simulink model "Monod_delay_Controller"  (R2020b)
settings: Solver=FixedStepAuto  StartTime=0.0  StopTime=constants.tend  FixedStep=constants.dt  RelTol=1e-3
undefined symbols (not defined in the file or in its folder): constants
libraries: pid_lib x2
settings Model: Creator=newpo  LastModifiedBy=newpo
settings DataIOCC: ReturnWorkspaceOutputs=off

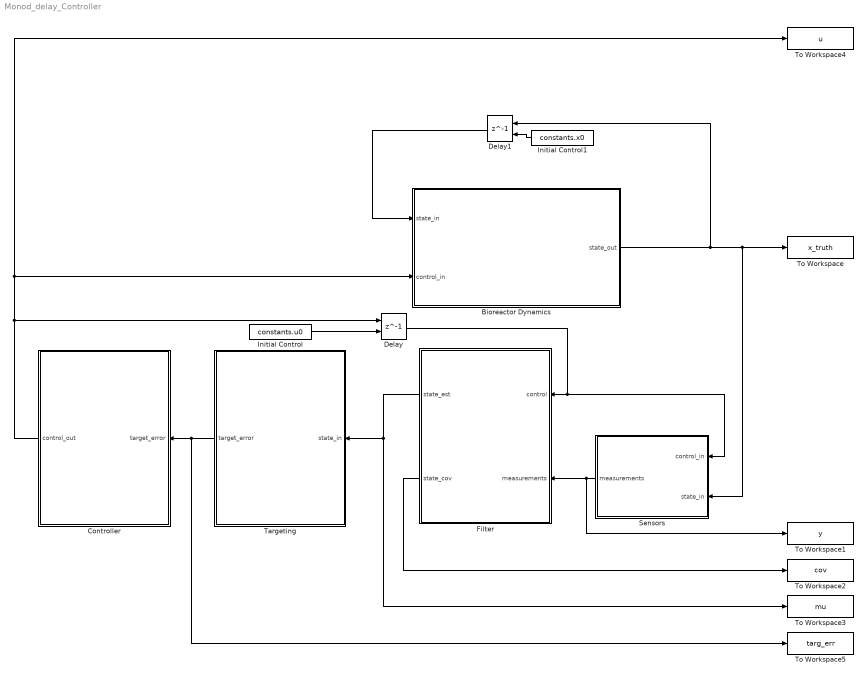
== system Monod_delay_Controller ==
  Bioreactor Dynamics : Subsystem
  Controller : Subsystem
  Delay : Delay  DelayLength=1  InitialConditionSource=Input port  InitialCondition=[constants.w;0;0;constants.Fg]
      settings: InputPortMap=u0,p4
  Delay1 : Delay  DelayLength=1  InitialConditionSource=Input port  InitialCondition=[constants.w;0;0;constants.Fg]
      settings: InputPortMap=u0,p4
  Filter : Subsystem
  Initial Control : Constant  Value=constants.u0
  Initial Control1 : Constant  Value=constants.x0
  Sensors : Subsystem
  Targeting : Subsystem
  To Workspace : ToWorkspace  VariableName=x_truth  SampleTime=-1
  To Workspace1 : ToWorkspace  VariableName=y  SampleTime=-1
  To Workspace2 : ToWorkspace  VariableName=cov  SampleTime=-1
  To Workspace3 : ToWorkspace  VariableName=mu  SampleTime=-1
  To Workspace4 : ToWorkspace  VariableName=u  SampleTime=-1
  To Workspace5 : ToWorkspace  VariableName=targ_err  SampleTime=-1
  wires:
  Bioreactor Dynamics/1(state_out) -> Delay1/1, Sensors/2(state_in), To Workspace/1
  Sensors/1(measurements) -> To Workspace1/1, Filter/2(measurements)
  Filter/1(state_est) -> To Workspace3/1, Targeting/1(state_in)
  Controller/1(control_out) -> To Workspace4/1, Bioreactor Dynamics/2(control_in), Delay/1
  Targeting/1(target_error) -> To Workspace5/1, Controller/1(target_error)
  Filter/2(state_cov) -> To Workspace2/1
  Delay/1 -> Sensors/1(control_in), Filter/1(control)
  Initial Control/1 -> Delay/2
  Delay1/1 -> Bioreactor Dynamics/1(state_in)
  Initial Control1/1 -> Delay1/2

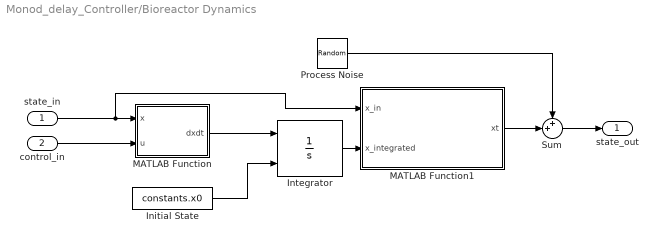
== system Monod_delay_Controller/Bioreactor Dynamics ==
  state_in : Inport
  control_in : Inport  Port=2
  Initial State : Constant  Value=constants.x0
  Integrator : Integrator  InitialConditionSource=external  LimitOutput=on  LowerSaturationLimit=0
  MATLAB Function : MATLAB Function  TreatAsAtomicUnit=on
  MATLAB Function1 : MATLAB Function  TreatAsAtomicUnit=on
  Process Noise : RandomNumber  Variance=diag(constants.Q)  SampleTime=constants.dt
  Sum : Sum  Inputs=++|
  state_out : Outport
  wires:
  Initial State/1 -> Integrator/2
  Sum/1 -> state_out/1
  Process Noise/1 -> Sum/1
  state_in/1 -> MATLAB Function1/1(x_in), MATLAB Function/1(x)
  control_in/1 -> MATLAB Function/2(u)
  MATLAB Function/1(dxdt) -> Integrator/1
  MATLAB Function1/1(xt) -> Sum/2
  Integrator/1 -> MATLAB Function1/2(x_integrated)

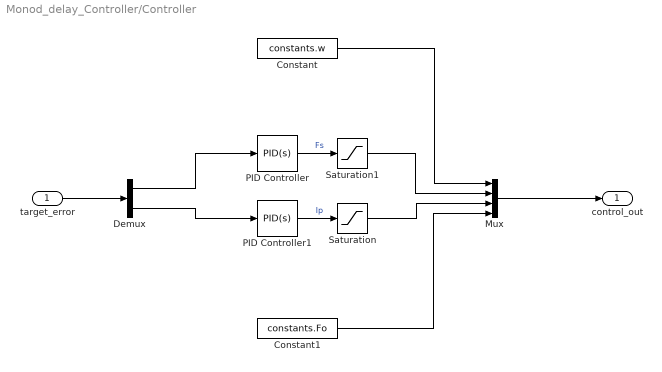
== system Monod_delay_Controller/Controller ==
  target_error : Inport
  Constant : Constant  Value=constants.w
  Constant1 : Constant  Value=constants.Fo
  Demux : Demux  Outputs=2
  Mux : Mux
  PID Controller : pid_lib/PID Controller  Controller=PID  Form=Parallel  TimeDomain=Continuous-time  UseExternalTs=off  SampleTime=-1  IntegratorMethod=Forward Euler  FilterMethod=Forward Euler  ControllerParametersSource=internal  P=constants.Fs_PID(1)  I=constants.Fs_PID(2)  D=constants.Fs_PID(3)  UseFilter=on  N=100  TunerSelectOption=Transfer Function Based (PID Tuner App)  InitialConditionSource=internal  InitialConditionForIntegrator=0  InitialConditionForFilter=0  DifferentiatorICPrevScaledInput=0  ExternalReset=none  TrackingMode=off  Kt=1  LimitOutput=off  SatLimitsSource=internal  UpperSaturationLimit=inf  LowerSaturationLimit=-inf  LinearizeAsGain=on  AntiWindupMode=none  Kb=1  POutMin=[]  POutMax=[]  IOutMin=[]  IOutMax=[]  DOutMin=[]  DOutMax=[]  NOutMin=[]  NOutMax=[]  SumOutMin=[]  SumOutMax=[]  SaturationOutMin=[]  SaturationOutMax=[]  PParamMin=[]  PParamMax=[]  IParamMin=[]  IParamMax=[]  DParamMin=[]  DParamMax=[]  NParamMin=[]  NParamMax=[]  KbParamMin=[]  KbParamMax=[]  KtParamMin=[]  KtParamMax=[]  KbOutMin=[]  KbOutMax=[]  KtOutMin=[]  KtOutMax=[]  IntegratorOutMin=[]  IntegratorOutMax=[]  FilterOutMin=[]  FilterOutMax=[]  SumI1OutMin=[]  SumI1OutMax=[]  SumI2OutMin=[]  SumI2OutMax=[]  SumI3OutMin=[]  SumI3OutMax=[]  SumI4OutMin=[]  SumI4OutMax=[]  SumDOutMin=[]  SumDOutMax=[]  DifferentiatorOutMin=[]  DifferentiatorOutMax=[]  FilterDiffOutCoefMin=[]  FilterDiffOutCoefMax=[]  ReciprocalOutMin=[]  ReciprocalOutMax=[]  SumDenOutMin=[]  SumDenOutMax=[]  SumNumOutMin=[]  SumNumOutMax=[]  DivideOutMin=[]  DivideOutMax=[]  UdiffTsProdOutMin=[]  UdiffTsProdOutMax=[]  NTsProdOutMin=[]  NTsProdOutMax=[]  UintegralTsProdOutMin=[]  UintegralTsProdOutMax=[]  UngainTsProdOutMin=[]  UngainTsProdOutMax=[]  IntegratorContinuousStateAttributes=''  IntegratorStateMustResolveToSignalObject=off  IntegratorRTWStateStorageClass=Auto  FilterContinuousStateAttributes=''  FilterStateMustResolveToSignalObject=off  FilterRTWStateStorageClass=Auto  ParallelPVariant=InternalParameters  IdealPVariant=Disabled  IVariant=InternalParameters  DVariant=InternalParameters  IntegratorVariant=Continuous  SatVariant=Disabled  AWVariant=Passthrough  PCopyVariant=Disabled  TRVariant=Disabled  FdbkBlocksVariant=Forward  IdealPFdbkVariant=Disabled  SatFdbkVariant=Disabled  DerivativeFilterVariant=ContFilter  NVariant=InternalParameters  NCopyVariant=Disabled  FilterICVariant=InternalICsFilter  IntegratorICVariant=InternalICs  ExternalResetVariant=Disabled  TRSumVariant=Passthrough  SumFdbkVariant=Disabled  SumVariant=Sum_PID  TsampFilterVariant=InternalTs  TsampNgainVariant=Passthrough  TsampIntegralVariant=Passthrough  ExternalSaturationOutDataTypeStr=Inherit: Same as second input
  PID Controller1 : pid_lib/PID Controller  Controller=PID  Form=Parallel  TimeDomain=Continuous-time  UseExternalTs=off  SampleTime=-1  IntegratorMethod=Forward Euler  FilterMethod=Forward Euler  ControllerParametersSource=internal  P=constants.IP_PID(1)  I=constants.IP_PID(2)  D=constants.IP_PID(3)  UseFilter=on  N=20  TunerSelectOption=Transfer Function Based (PID Tuner App)  InitialConditionSource=internal  InitialConditionForIntegrator=0  InitialConditionForFilter=0  DifferentiatorICPrevScaledInput=0  ExternalReset=none  TrackingMode=off  Kt=1  LimitOutput=off  SatLimitsSource=internal  UpperSaturationLimit=inf  LowerSaturationLimit=-inf  LinearizeAsGain=on  AntiWindupMode=none  Kb=1  POutMin=[]  POutMax=[]  IOutMin=[]  IOutMax=[]  DOutMin=[]  DOutMax=[]  NOutMin=[]  NOutMax=[]  SumOutMin=[]  SumOutMax=[]  SaturationOutMin=[]  SaturationOutMax=[]  PParamMin=[]  PParamMax=[]  IParamMin=[]  IParamMax=[]  DParamMin=[]  DParamMax=[]  NParamMin=[]  NParamMax=[]  KbParamMin=[]  KbParamMax=[]  KtParamMin=[]  KtParamMax=[]  KbOutMin=[]  KbOutMax=[]  KtOutMin=[]  KtOutMax=[]  IntegratorOutMin=[]  IntegratorOutMax=[]  FilterOutMin=[]  FilterOutMax=[]  SumI1OutMin=[]  SumI1OutMax=[]  SumI2OutMin=[]  SumI2OutMax=[]  SumI3OutMin=[]  SumI3OutMax=[]  SumI4OutMin=[]  SumI4OutMax=[]  SumDOutMin=[]  SumDOutMax=[]  DifferentiatorOutMin=[]  DifferentiatorOutMax=[]  FilterDiffOutCoefMin=[]  FilterDiffOutCoefMax=[]  ReciprocalOutMin=[]  ReciprocalOutMax=[]  SumDenOutMin=[]  SumDenOutMax=[]  SumNumOutMin=[]  SumNumOutMax=[]  DivideOutMin=[]  DivideOutMax=[]  UdiffTsProdOutMin=[]  UdiffTsProdOutMax=[]  NTsProdOutMin=[]  NTsProdOutMax=[]  UintegralTsProdOutMin=[]  UintegralTsProdOutMax=[]  UngainTsProdOutMin=[]  UngainTsProdOutMax=[]  IntegratorContinuousStateAttributes=''  IntegratorStateMustResolveToSignalObject=off  IntegratorRTWStateStorageClass=Auto  FilterContinuousStateAttributes=''  FilterStateMustResolveToSignalObject=off  FilterRTWStateStorageClass=Auto  ParallelPVariant=InternalParameters  IdealPVariant=Disabled  IVariant=InternalParameters  DVariant=InternalParameters  IntegratorVariant=Continuous  SatVariant=Disabled  AWVariant=Passthrough  PCopyVariant=Disabled  TRVariant=Disabled  FdbkBlocksVariant=Forward  IdealPFdbkVariant=Disabled  SatFdbkVariant=Disabled  DerivativeFilterVariant=ContFilter  NVariant=InternalParameters  NCopyVariant=Disabled  FilterICVariant=InternalICsFilter  IntegratorICVariant=InternalICs  ExternalResetVariant=Disabled  TRSumVariant=Passthrough  SumFdbkVariant=Disabled  SumVariant=Sum_PID  TsampFilterVariant=InternalTs  TsampNgainVariant=Passthrough  TsampIntegralVariant=Passthrough  ExternalSaturationOutDataTypeStr=Inherit: Same as second input
  Saturation : Saturate  UpperLimit=constants.Ip_max  LowerLimit=-constants.Ip_max
  Saturation1 : Saturate  UpperLimit=constants.Fs_max  LowerLimit=0
  control_out : Outport
  wires:
  Mux/1 -> control_out/1
  target_error/1 -> Demux/1
  PID Controller/1 -> Saturation1/1  "Fs"
  Demux/1 -> PID Controller/1
  Constant/1 -> Mux/1
  Constant1/1 -> Mux/4
  PID Controller1/1 -> Saturation/1  "Ip"
  Demux/2 -> PID Controller1/1
  Saturation/1 -> Mux/3
  Saturation1/1 -> Mux/2

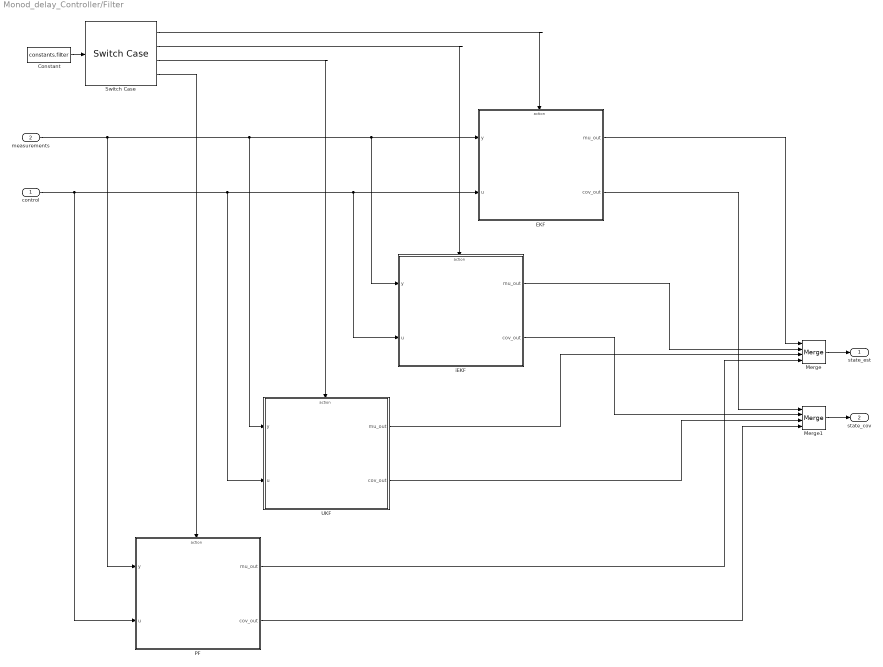
== system Monod_delay_Controller/Filter ==
  control : Inport
  measurements : Inport  Port=2
  Constant : Constant  Value=constants.filter
  EKF : Subsystem  TreatAsAtomicUnit=on
  Merge : Merge  Inputs=4
  Merge1 : Merge  Inputs=4
  PF : Subsystem  TreatAsAtomicUnit=on
  Switch Case : SwitchCase  CaseConditions={FilterTypes.EKF,FilterTypes.iEKF,FilterTypes.UKF,FilterTypes.PF}  ShowDefaultCase=off
  UKF : Subsystem  TreatAsAtomicUnit=on
  iEKF : Subsystem  TreatAsAtomicUnit=on
  state_est : Outport
  state_cov : Outport  Port=2
  wires:
  measurements/1 -> PF/1(y), UKF/1(y), EKF/1(y), iEKF/1(y)
  control/1 -> PF/2(u), UKF/2(u), EKF/2(u), iEKF/2(u)
  EKF/2(cov_out) -> Merge1/1
  Switch Case/1 -> EKF/Action
  Switch Case/2 -> iEKF/Action
  EKF/1(mu_out) -> Merge/1
  iEKF/1(mu_out) -> Merge/2
  Merge/1 -> state_est/1
  Merge1/1 -> state_cov/1
  iEKF/2(cov_out) -> Merge1/2
  Constant/1 -> Switch Case/1
  Switch Case/3 -> UKF/Action
  UKF/1(mu_out) -> Merge/3
  UKF/2(cov_out) -> Merge1/3
  Switch Case/4 -> PF/Action
  PF/2(cov_out) -> Merge1/4
  PF/1(mu_out) -> Merge/4

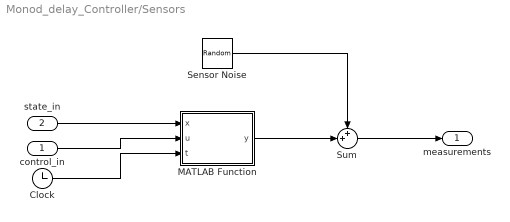
== system Monod_delay_Controller/Sensors ==
  control_in : Inport
  state_in : Inport  Port=2
  Clock : Clock
  MATLAB Function : MATLAB Function  TreatAsAtomicUnit=on
  Sensor Noise : RandomNumber  Variance=diag(constants.R)  SampleTime=constants.dt
  Sum : Sum  Inputs=++|
  measurements : Outport
  wires:
  state_in/1 -> MATLAB Function/1(x)
  control_in/1 -> MATLAB Function/2(u)
  MATLAB Function/1(y) -> Sum/2
  Sum/1 -> measurements/1
  Sensor Noise/1 -> Sum/1
  Clock/1 -> MATLAB Function/3(t)

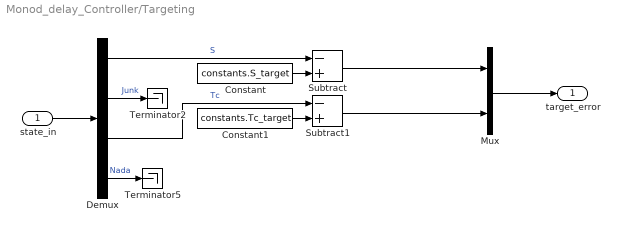
== system Monod_delay_Controller/Targeting ==
  state_in : Inport
  Constant : Constant  Value=constants.S_target
  Constant1 : Constant  Value=constants.Tc_target
  Demux : Demux  Outputs=[1 2 1 -1]
  Mux : Mux  Inputs=2
  Subtract : Sum  Inputs=-+
  Subtract1 : Sum  Inputs=-+
  Terminator2 : Terminator
  Terminator5 : Terminator
  target_error : Outport
  wires:
  state_in/1 -> Demux/1
  Demux/1 -> Subtract/1  "S"
  Constant/1 -> Subtract/2
  Constant1/1 -> Subtract1/2
  Subtract/1 -> Mux/1
  Subtract1/1 -> Mux/2
  Mux/1 -> target_error/1
  Demux/2 -> Terminator2/1  "Junk"
  Demux/4 -> Terminator5/1  "Nada"
  Demux/3 -> Subtract1/1  "Tc"

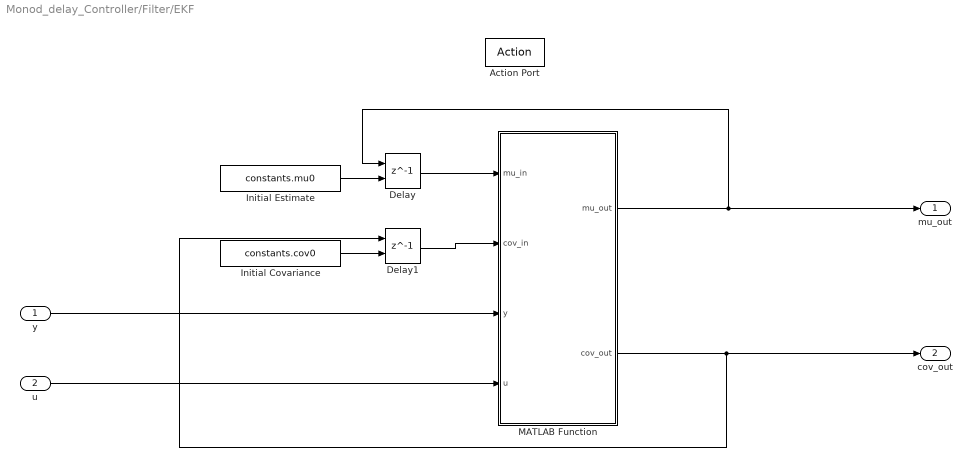
== system Monod_delay_Controller/Filter/EKF ==
  y : Inport
  u : Inport  Port=2
  Action Port : ActionPort  ActionPortLabel=case [ EKF ]:
  Delay : Delay  DelayLength=1  InitialConditionSource=Input port  InitialCondition=0
      settings: InputPortMap=u0,p4
  Delay1 : Delay  DelayLength=1  InitialConditionSource=Input port  InitialCondition=0
      settings: InputPortMap=u0,p4
  Initial Covariance : Constant  Value=constants.cov0
  Initial Estimate : Constant  Value=constants.mu0
  MATLAB Function : MATLAB Function  TreatAsAtomicUnit=on
  mu_out : Outport
  cov_out : Outport  Port=2
  wires:
  y/1 -> MATLAB Function/3(y)
  Initial Estimate/1 -> Delay/2
  Delay1/1 -> MATLAB Function/2(cov_in)
  MATLAB Function/2(cov_out) -> cov_out/1, Delay1/1
  Initial Covariance/1 -> Delay1/2
  u/1 -> MATLAB Function/4(u)
  MATLAB Function/1(mu_out) -> mu_out/1, Delay/1
  Delay/1 -> MATLAB Function/1(mu_in)

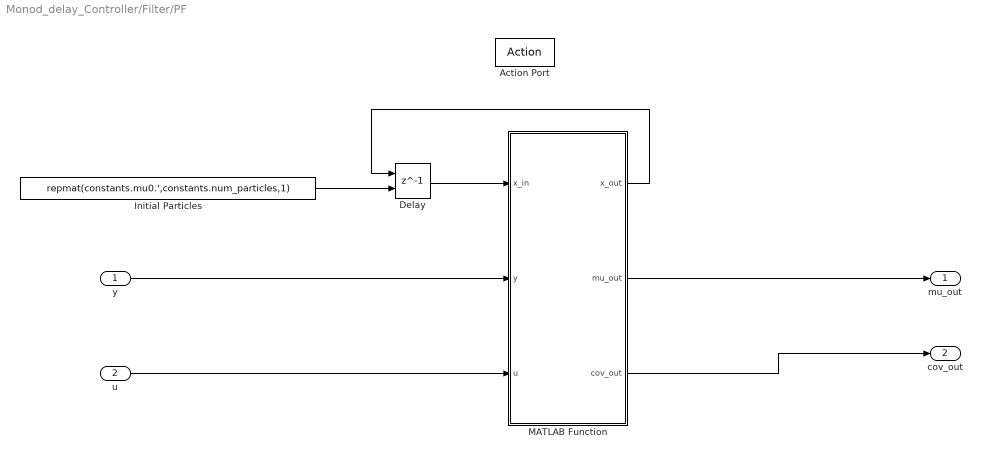
== system Monod_delay_Controller/Filter/PF ==
  y : Inport
  u : Inport  Port=2
  Action Port : ActionPort  ActionPortLabel=case [ PF ]:
  Delay : Delay  DelayLength=1  InitialConditionSource=Input port  InitialCondition=0
      settings: InputPortMap=u0,p4
  Initial Particles : Constant  Value=repmat(constants.mu0.',constants.num_particles,1)
  MATLAB Function : MATLAB Function  TreatAsAtomicUnit=on
  mu_out : Outport
  cov_out : Outport  Port=2
  wires:
  y/1 -> MATLAB Function/2(y)
  MATLAB Function/3(cov_out) -> cov_out/1
  u/1 -> MATLAB Function/3(u)
  MATLAB Function/2(mu_out) -> mu_out/1
  Delay/1 -> MATLAB Function/1(x_in)
  MATLAB Function/1(x_out) -> Delay/1
  Initial Particles/1 -> Delay/2

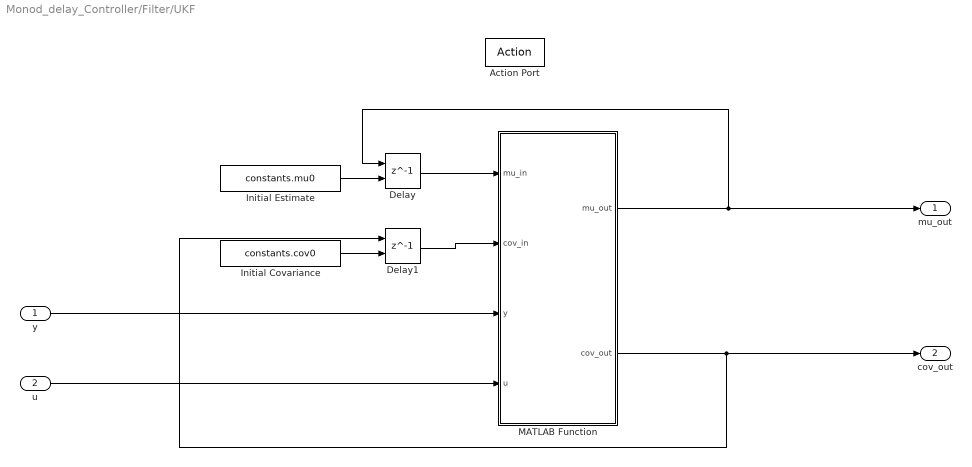
== system Monod_delay_Controller/Filter/UKF ==
  y : Inport
  u : Inport  Port=2
  Action Port : ActionPort  ActionPortLabel=case [ UKF ]:
  Delay : Delay  DelayLength=1  InitialConditionSource=Input port  InitialCondition=0
      settings: InputPortMap=u0,p4
  Delay1 : Delay  DelayLength=1  InitialConditionSource=Input port  InitialCondition=0
      settings: InputPortMap=u0,p4
  Initial Covariance : Constant  Value=constants.cov0
  Initial Estimate : Constant  Value=constants.mu0
  MATLAB Function : MATLAB Function  TreatAsAtomicUnit=on
  mu_out : Outport
  cov_out : Outport  Port=2
  wires:
  y/1 -> MATLAB Function/3(y)
  Initial Estimate/1 -> Delay/2
  Delay1/1 -> MATLAB Function/2(cov_in)
  MATLAB Function/2(cov_out) -> cov_out/1, Delay1/1
  Initial Covariance/1 -> Delay1/2
  u/1 -> MATLAB Function/4(u)
  MATLAB Function/1(mu_out) -> mu_out/1, Delay/1
  Delay/1 -> MATLAB Function/1(mu_in)

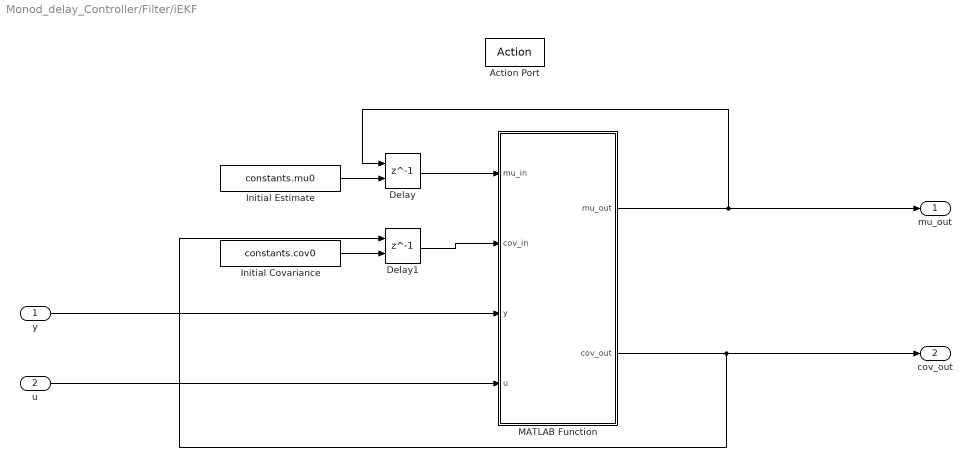
== system Monod_delay_Controller/Filter/iEKF ==
  y : Inport
  u : Inport  Port=2
  Action Port : ActionPort  ActionPortLabel=case [ iEKF ]:
  Delay : Delay  DelayLength=1  InitialConditionSource=Input port  InitialCondition=0
      settings: InputPortMap=u0,p4
  Delay1 : Delay  DelayLength=1  InitialConditionSource=Input port  InitialCondition=0
      settings: InputPortMap=u0,p4
  Initial Covariance : Constant  Value=constants.cov0
  Initial Estimate : Constant  Value=constants.mu0
  MATLAB Function : MATLAB Function  TreatAsAtomicUnit=on
  mu_out : Outport
  cov_out : Outport  Port=2
  wires:
  y/1 -> MATLAB Function/3(y)
  Initial Estimate/1 -> Delay/2
  Delay1/1 -> MATLAB Function/2(cov_in)
  MATLAB Function/2(cov_out) -> cov_out/1, Delay1/1
  Initial Covariance/1 -> Delay1/2
  u/1 -> MATLAB Function/4(u)
  MATLAB Function/1(mu_out) -> mu_out/1, Delay/1
  Delay/1 -> MATLAB Function/1(mu_in)

== matlab function Monod_delay_Controller/Filter/iEKF/MATLAB Function ==
  data: mu_in input; cov_in input; y input; u input; mu_out output; cov_out output; constants parameter
function [mu_out, cov_out] = Monod_iEKF(mu_in, cov_in, y, u, constants)
    % Collect inputs
%     S = mu_in(1); % cell concentration, g/l
%     C = mu_in(2); % substrate concentration, g/l
%     QO2 = mu_in(3); % OTR = OUR, moles/sec
%     Tc = mu_in(4); % Temperature of culture
%     Tinf = mu_in(5); % Temperature of environment
%     V = mu_in(6); % Volume of tank
    mygrowthrate = mu(mu_in(1),mu_in(2)); 
    
    % Collect controls
    w = u(1); % agitator speed, rpm
    Fs = u(2); % substrate feed rate, L/s
    Ip = u(3); % Peltier current, amps
    Fg = u(4); % air feed rate, SLPS
    kLa = w^(1.7)/(Fg^0.1); % kLa coeff
    
    % Collect measurements
%     mf_out = y(1);
%     DO = y(2);
%     Tc_meas = y(3);
%     Tinf_meas = y(4);

    y_end = length(y);
    if y(end) < -1
       y_end = 5; 
    end
    
    % EKF Update
    mu_p = f(mu_in);
    At = A(mu_in);
    cov_p = At*cov_in*(At.') + constants.Q;
    
    % iEKF iteration
    iter_max = 2500; % max number of iterations
    tol = 1E-5;
    n = 0;
    mu_pred = mu_p; % hold the original prediction step mean
    mu_i = mu_p;
    while n < iter_max
        % calculate matrices from previous state
        Ct = C(mu_i); Ct = Ct(1:y_end,:); % update using last time step
        Kt = cov_p*(Ct.')/(Ct*cov_p*(Ct.')+constants.R(1:y_end,1:y_end)); % Kalman gain, using new Ct
        z = g(mu_i);
        z = y(1:y_end) - z(1:y_end);
        mu_i = mu_pred + Kt*(z + Ct*(mu_i - mu_pred));
        err = norm(mu_i - mu_p);
        if err < tol % check convergence between previous step and updated
            break;
        end
        mu_p = mu_i;
        n = n + 1;
    end
    
    Ct = C(mu_i); Ct = Ct(1:y_end,:);
    Kt = cov_p*(Ct.')/(Ct*cov_p*(Ct.')+constants.R(1:y_end,1:y_end)); % Kalman gain
    mu_out = mu_i;
    cov_out = (eye(length(mu_in)) - Kt*Ct)*cov_p;
    
    function xt = f(x)
       xt = zeros(size(x));
       
       xt(1) = x(1) + constants.dt*((constants.S0-x(1))*Fs/x(6)- mygrowthrate/constants.Yxs - constants.m*x(2)); % S = substrate conc
       xt(2) = x(2) + constants.dt*(-Fs/x(6)*x(2)+mygrowthrate); % C = cell conc
       xt(3) = x(3); % QO2 = OUR coefficient
       xt(4) = x(4) + constants.dt/constants.C_heat/x(6)*(constants.N_power*(w^3)+constants.Kq*x(3)*x(2)+(constants.Pp*Ip+(Ip^2)*constants.Rp)*constants.Np + constants.hA*(x(4)-x(5))); % Tc = culture temp
       xt(5) = x(5); % Tinf = environment temp
       xt(6) = x(6) + constants.dt*Fs;
       xt(7:8) = x(1:2);
       if constants.sample_interval > 1
           for i = 2:constants.sample_interval 
               xt(2*i+5:2*i+6) = x(2*i+3:2*i+4); % delayed states
           end
       end
    end
    function At = A(x)
        At = zeros(length(x));
        mymu = mu(x(1),x(2));
        dmu = constants.mu_max*x(2)*constants.Ki*(constants.Ki*constants.Ks-(x(1)^2))/((constants.Ki+x(1))^2)/((constants.Ks+x(1))^2);
        At(1,1) = 1 + constants.dt*(-Fs/x(6)-dmu/constants.Yxs);
        At(1,2) = -constants.dt*mymu - constants.m;
        At(1,6) = -constants.dt*(constants.S0-x(1))*Fs/(x(6)^2);
        At(2,1) = constants.dt*(-Fs/x(6) + dmu);
        At(2,2) = 1 - constants.dt*Fs/x(6) + constants.dt*mymu ;
        At(2,6) = constants.dt*Fs*x(2)/(x(6)^2);
        At(3,3) = 1;
        At(4,2) = constants.dt/constants.C_heat/x(6)*constants.Kq*x(3);
        At(4,3) = constants.dt/constants.C_heat/x(6)*constants.Kq*x(2);
        At(4,4) = 1 + constants.dt/constants.C_heat/x(6)*constants.hA;
        At(4,5) = -constants.dt/constants.C_heat/x(6)*constants.hA;
        At(4,6) = -constants.dt/constants.C_heat/(x(6)^2)*(constants.N_power*(w^3)+constants.Kq*x(3)*x(2)+(constants.Pp*Ip+(Ip^2)*constants.Rp)*constants.Np + constants.hA*(x(4)-x(5))); 
        At(5,5) = 1;
        At(6,6) = 1;
        At(7:8,1:2) = eye(2);
        if constants.sample_interval > 1
           for i = 2:constants.sample_interval 
               At(2*i+5:2*i+6,2*i+3:2*i+4) = eye(2); % delayed states
           end
        end
    end
    function ypred = g(x)
        ypred = zeros(length(y),1);
        ypred(1) = constants.mf_in - x(3)*x(2)/Fg; % Measured mass fraction of O2 leaving system
        ypred(2) = 1 - 1/constants.mf_in*(1/Fg - 1/kLa/constants.pr)*x(3)*x(2); % Measured DO2
        ypred(3) = x(4); % Measured Tc
        ypred(4) = x(5); % measured Tinf
        ypred(5) = x(6);  % measured volume
        ypred(6:7) = x(end-1:end); % last two items in x are the most delayed
    end
    function Ct = C(x)
       Ct = zeros(length(y),length(x));
       Ct(1,2) = -x(3)/Fg;
       Ct(1,3) = -x(2)/Fg;
       Ct(2,2) = -1/constants.mf_in * (1/Fg - 1/constants.pr/kLa)*x(3);
       Ct(2,3) = -1/constants.mf_in * (1/Fg - 1/constants.pr/kLa)*x(2);
       Ct(3,4) = 1;
       Ct(4,5) = 1;
       Ct(5,6) = 1;
       Ct(6,end-1) = 1; % last two items in x are the most delayed
       Ct(7,end) = 1;
    end
    function mut = mu(S,C)
        mut = constants.mu_max*constants.Ki*S/(constants.Ki+S)/(constants.Ks+S)*C ;
    end
end

== matlab function Monod_delay_Controller/Bioreactor Dynamics/MATLAB Function ==
  data: x input; u input; dxdt output; constants parameter
function dxdt = statedot(x,u,constants)
    dxdt = zeros(size(x));
    w = u(1); % agitator speed
    Fs = u(2); % substrate feed rate
    Ip = u(3); % Peltier currents
    mu = constants.mu_max*x(2)*constants.Ki*x(1)/(constants.Ki+x(1))/(constants.Ks+x(1));
    dxdt(1) = constants.S0*Fs/x(6) - Fs/x(6)*x(1) - mu/constants.Yxs - constants.m*x(2); % S = substrate conc
    dxdt(2) = -Fs/x(6)*x(2) + mu; % C = cell conc
    dxdt(3) = 0; % QO2 = OUR coefficient
    dxdt(4) = 1/constants.C_heat/x(6)*(constants.N_power*(w^3)+constants.Kq*x(3)*x(2)+(constants.Pp*Ip+(Ip^2)*constants.Rp)*constants.Np + constants.hA*(x(4)-x(5))); % Tc = culture temp
    dxdt(5) = 0; % Tinf = environment temp
    dxdt(6) = Fs;
    dxdt(7:end) = 0; % these are updated after integration
end

== matlab function Monod_delay_Controller/Sensors/MATLAB Function ==
  data: x input; u input; t input; y output; constants parameter
function y = g(x,u,t,constants)
    y = zeros(7,1);
    w = u(1);
    Fg = u(4);
    kLa = (w^1.7)/(Fg^0.1);
    y(1) = constants.mf_in - x(3)*x(2)/Fg; % Measured mass fraction of O2 leaving system
    y(2) = 1 - 1/constants.mf_in*(1/Fg - 1/kLa/constants.pr)*x(3)*x(2); % Measured DO2
    y(3) = x(4); % Measured Tc
    y(4) = x(5); % measured Tinf
    y(5) = x(6); % measured volume
    if floor(t/constants.dt) > 0 && mod(floor(t/constants.dt),constants.sample_interval)==0
       y(6:7) = x(end-1:end); % last two measurements are delayed by sample_interval
    else
       y(6:7) = [-100; -100]; % throw in bullshit to indicate no major sample 
    end
end

== matlab function Monod_delay_Controller/Filter/EKF/MATLAB Function ==
  data: mu_in input; cov_in input; y input; u input; mu_out output; cov_out output; constants parameter
function [mu_out, cov_out] = Monod_EKF(mu_in, cov_in, y, u, constants)
    % Collect inputs
%     S = mu_in(1); % cell concentration, g/l
%     C = mu_in(2); % substrate concentration, g/l
%     QO2 = mu_in(3); % OTR = OUR, moles/sec
%     Tc = mu_in(4); % Temperature of culture
%     Tinf = mu_in(5); % Temperature of environment
%     V = mu_in(6); % Volume of tank
    mygrowthrate = mu(mu_in(1),mu_in(2)); 
    
    % Collect controls
    w = u(1); % agitator speed, rpm
    Fs = u(2); % substrate feed rate, L/s
    Ip = u(3); % Peltier current, amps
    Fg = u(4); % air feed rate, SLPS
    kLa = w^(1.7)/(Fg^0.1); % kLa coeff
    
    % Collect measurements
%     mf_out = y(1);
%     DO = y(2);
%     Tc_meas = y(3);
%     Tinf_meas = y(4);

    y_end = length(y);
    if y(end) < -1
       y_end = 5; 
    end
    
    % EKF Update
    mu_p = f(mu_in);
    At = A(mu_in);
    cov_p = At*cov_in*(At.') + constants.Q;
    
    % EKF Prediction
    Ct = C(mu_p); Ct = Ct(1:y_end,:);
    ypred = g(mu_p); ypred = ypred(1:y_end);
    Kt = cov_p*(Ct.')/(Ct*cov_p*(Ct.')+constants.R(1:y_end,1:y_end)); % Kalman gain
    mu_out = mu_p + Kt*(y(1:y_end) - ypred);
    cov_out = (eye(length(mu_in)) - Kt*Ct)*cov_p;
    
    function xt = f(x)
       xt = zeros(size(x));
       
       xt(1) = x(1) + constants.dt*((constants.S0-x(1))*Fs/x(6)- mygrowthrate/constants.Yxs - constants.m*x(2)); % S = substrate conc
       xt(2) = x(2) + constants.dt*(-Fs/x(6)*x(2)+mygrowthrate); % C = cell conc
       xt(3) = x(3); % QO2 = OUR coefficient
       xt(4) = x(4) + constants.dt/constants.C_heat/x(6)*(constants.N_power*(w^3)+constants.Kq*x(3)*x(2)+(constants.Pp*Ip+(Ip^2)*constants.Rp)*constants.Np + constants.hA*(x(4)-x(5))); % Tc = culture temp
       xt(5) = x(5); % Tinf = environment temp
       xt(6) = x(6) + constants.dt*Fs;
       xt(7:8) = x(1:2);
       if constants.sample_interval > 1
           for i = 2:constants.sample_interval 
               xt(2*i+5:2*i+6) = x(2*i+3:2*i+4); % delayed states
           end
       end
    end
    function At = A(x)
        At = zeros(length(x));
        mymu = mu(x(1),x(2));
        dmu = constants.mu_max*x(2)*constants.Ki*(constants.Ki*constants.Ks-(x(1)^2))/((constants.Ki+x(1))^2)/((constants.Ks+x(1))^2);
        At(1,1) = 1 + constants.dt*(-Fs/x(6)-dmu/constants.Yxs);
        At(1,2) = -constants.dt*mymu - constants.m;
        At(1,6) = -constants.dt*(constants.S0-x(1))*Fs/(x(6)^2);
        At(2,1) = constants.dt*(-Fs/x(6) + dmu);
        At(2,2) = 1 - constants.dt*Fs/x(6) + constants.dt*mymu ;
        At(2,6) = constants.dt*Fs*x(2)/(x(6)^2);
        At(3,3) = 1;
        At(4,2) = constants.dt/constants.C_heat/x(6)*constants.Kq*x(3);
        At(4,3) = constants.dt/constants.C_heat/x(6)*constants.Kq*x(2);
        At(4,4) = 1 + constants.dt/constants.C_heat/x(6)*constants.hA;
        At(4,5) = -constants.dt/constants.C_heat/x(6)*constants.hA;
        At(4,6) = -constants.dt/constants.C_heat/(x(6)^2)*(constants.N_power*(w^3)+constants.Kq*x(3)*x(2)+(constants.Pp*Ip+(Ip^2)*constants.Rp)*constants.Np + constants.hA*(x(4)-x(5))); 
        At(5,5) = 1;
        At(6,6) = 1;
        At(7:8,1:2) = eye(2);
        if constants.sample_interval > 1
           for i = 2:constants.sample_interval 
               At(2*i+5:2*i+6,2*i+3:2*i+4) = eye(2); % delayed states
           end
        end
    end
    function ypred = g(x)
        ypred = zeros(length(y),1);
        ypred(1) = constants.mf_in - x(3)*x(2)/Fg; % Measured mass fraction of O2 leaving system
        ypred(2) = 1 - 1/constants.mf_in*(1/Fg - 1/kLa/constants.pr)*x(3)*x(2); % Measured DO2
        ypred(3) = x(4); % Measured Tc
        ypred(4) = x(5); % measured Tinf
        ypred(5) = x(6);  % measured volume
        ypred(6:7) = x(end-1:end); % last two items in x are the most delayed
    end
    function Ct = C(x)
       Ct = zeros(length(y),length(x));
       Ct(1,2) = -x(3)/Fg;
       Ct(1,3) = -x(2)/Fg;
       Ct(2,2) = -1/constants.mf_in * (1/Fg - 1/constants.pr/kLa)*x(3);
       Ct(2,3) = -1/constants.mf_in * (1/Fg - 1/constants.pr/kLa)*x(2);
       Ct(3,4) = 1;
       Ct(4,5) = 1;
       Ct(5,6) = 1;
       Ct(6,end-1) = 1; % last two items in x are the most delayed
       Ct(7,end) = 1;
    end
    function mut = mu(S,C)
        mut = constants.mu_max*constants.Ki*S/(constants.Ki+S)/(constants.Ks+S)*C ;
    end
end

== matlab function Monod_delay_Controller/Filter/UKF/MATLAB Function ==
  data: mu_in input; cov_in input; y input; u input; mu_out output; cov_out output; constants parameter
function [mu_out, cov_out] = Monod_UKF(mu_in, cov_in, y, u, constants)
    % Collect inputs
%     S = mu_in(1); % cell concentration, g/l
%     C = mu_in(2); % substrate concentration, g/l
%     QO2 = mu_in(3); % OTR = OUR, moles/sec
%     Tc = mu_in(4); % Temperature of culture
%     Tinf = mu_in(5); % Temperature of environment
%     V = mu_in(6); % Volume of tank
    
    y_end = length(y);
    if y(end) < -1
       y_end = 5; 
    end

    % Collect controls
    w = u(1); % agitator speed, rpm
    Fs = u(2); % substrate feed rate, L/s
    Ip = u(3); % Peltier current, amps
    Fg = u(4); % air feed rate, SLPS
    kLa = w^(1.7)/(Fg^0.1); % kLa coeff
    
    % Collect measurements
%     mf_out = y(1);
%     DO = y(2);
%     Tc_meas = y(3);
%     Tinf_meas = y(4);

    lambda=2;
    n = length(mu_in);
    weights = zeros(2*length(mu_in)+1,1);
    weights(1) = lambda/(lambda+length(mu_in));
    weights(2:2*n+1) = 0.5/(lambda+n);
   %% UKF Predict 
   xlast = sig_point(mu_in,cov_in);
   xbar = zeros(2*length(mu_in)+1,length(mu_in));
   for j = 1:(2*n+1)
       xbar(j,:) = f(xlast(j,:).');
   end
   [mu_p, cov_p] = sig_inv(xbar, weights, constants.Q);
   %% UKF Update
   xnew = sig_point(mu_p, cov_p);
   yi = zeros(2*length(mu_in)+1,y_end);
   for j = 1:(2*n+1)
       z = g(xnew(j,:).');
       yi(j,:) = z(1:y_end);
   end
   yhat = sum((weights*ones(1,y_end)).*yi, 1).'; % weighted sum of columns
   covy = constants.R(1:y_end,1:y_end);
   covxy = zeros(length(mu_in),y_end);
   for j = 1:2*n+1
       covy = covy + weights(j)*(yi(j,:).' - yhat)*(yi(j,:)-yhat.');
       covxy = covxy + weights(j)*(xnew(j,:).' - mu_p)*(yi(j,:)-yhat.');
   end
   covy = inv(covy);
   mu_out = mu_p + covxy*covy*(y(1:y_end) - yhat);
   cov_out = cov_p - covxy*covy*(covxy.');
    
   %% Helper functions
   function x = sig_point(m, sig)
       x = zeros(2*length(mu_in) + 1, length(m));
       x(1,:) = m;
       [U,S,~] = svd(sig); % SVD method for matrix sqrt
       M = U*sqrt(S)*(U.'); % primary axis aligned
       for k = 2:(2*n+1)
           x(k,:) = m + (1-2*mod(k,2))*sqrt(n+lambda)*M(:,floor(k/2));
       end
    end

    function [m, sig] = sig_inv(x, w, Q)
       m = sum((w*ones(1,length(mu_in))).*x).'; 
       sig = Q ;
       for k = 1:(2*n+1)
           sig = sig + w(k)*(x(k,:).'-m)*(x(k,:)-m.');
       end
    end
    
    function xt = f(x)
       xt = zeros(size(x));
       mygrowthrate = mu(x(1),x(2));
       xt(1) = x(1) + constants.dt*((constants.S0-x(1))*Fs/x(6)- mygrowthrate/constants.Yxs - constants.m*x(2)); % S = substrate conc
       xt(2) = x(2) + constants.dt*(-Fs/x(6)*x(2)+mygrowthrate); % C = cell conc
       xt(3) = x(3); % QO2 = OUR coefficient
       xt(4) = x(4) + constants.dt/constants.C_heat/x(6)*(constants.N_power*(w^3)+constants.Kq*x(3)*x(2)+(constants.Pp*Ip+(Ip^2)*constants.Rp)*constants.Np + constants.hA*(x(4)-x(5))); % Tc = culture temp
       xt(5) = x(5); % Tinf = environment temp
       xt(6) = x(6) + constants.dt*Fs;
       xt(7:8) = x(1:2);
       if constants.sample_interval > 1
           for i = 2:constants.sample_interval 
               xt(2*i+5:2*i+6) = x(2*i+3:2*i+4); % delayed states
           end
       end
    end

    function ypred = g(x)
        ypred = zeros(length(y),1);
        ypred(1) = constants.mf_in - x(3)*x(2)/Fg; % Measured mass fraction of O2 leaving system
        ypred(2) = 1 - 1/constants.mf_in*(1/Fg - 1/kLa/constants.pr)*x(3)*x(2); % Measured DO2
        ypred(3) = x(4); % Measured Tc
        ypred(4) = x(5); % measured Tinf
        ypred(5) = x(6);  % measured volume
        ypred(6:7) = x(end-1:end); % last two items in x are the most delayed
    end

    function mut = mu(S,C)
        mut = constants.mu_max*constants.Ki*S/(constants.Ki+S)/(constants.Ks+S)*C ;
    end
end

== matlab function Monod_delay_Controller/Filter/PF/MATLAB Function ==
  data: x_out output; x_in input; y input; u input; mu_out output; cov_out output; constants parameter
function [x_out, mu_out, cov_out] = Monod_PF(x_in, y, u, constants)
    % Collect inputs
%     S = mu_in(1); % cell concentration, g/l
%     C = mu_in(2); % substrate concentration, g/l
%     QO2 = mu_in(3); % OTR = OUR, moles/sec
%     Tc = mu_in(4); % Temperature of culture
%     Tinf = mu_in(5); % Temperature of environment
%     V = mu_in(6); % Volume of tank
    
    % Collect controls
    w = u(1); % agitator speed, rpm
    Fs = u(2); % substrate feed rate, L/s
    Ip = u(3); % Peltier current, amps
    Fg = u(4); % air feed rate, SLPS
    kLa = w^(1.7)/(Fg^0.1); % kLa coeff
    
    % Collect measurements
%     mf_out = y(1);
%     DO = y(2);
%     Tc_meas = y(3);
%     Tinf_meas = y(4);

    y_end = length(y);
    if y(end) < -1
       y_end = 5; 
    end

    N = constants.num_particles; % number of particles
    n = size(x_in,2);
    x_p = zeros(size(x_in));
    ws = zeros(N,1);
    %% PF Update
    for i = 1:N
        x_p(i,:) = f(x_in(i,:).') + sqrt(constants.Q)*randn(n,1);
        z = g(x_p(i,:).');
        z = y(1:y_end) - z(1:y_end);
        ws(i) = gaussian_val(z, constants.R(1:y_end,1:y_end));
    end
    ws = ws/sum(ws);
    
    %% PF Predict
    edges = [0; cumsum(ws)];
    s = rand(size(x_in,1),1);
    bins = discretize(s,edges);
    x_out = x_p(bins,:);
    
    %% Compute mean and cov
    mu_out = sum((ws*ones(1,n)).*x_out, 1).';
    cov_out = zeros(size(x_in,2));
    for k= 1:N
       diff = (x_out(k,:)-mu_out.');
       cov_out = cov_out + ws(k)*(diff.') * diff;
    end
    
   %% Helper functions
    function p = gaussian_val(x,cov)
       p = 1/sqrt((2*pi)^n * det(cov)) * exp(-0.5*(x.')*(cov\x));
    end
    
    function xt = f(x)
       xt = zeros(size(x));
       mygrowthrate = mu(x(1),x(2));
       xt(1) = x(1) + constants.dt*((constants.S0-x(1))*Fs/x(6)- mygrowthrate/constants.Yxs - constants.m*x(2)); % S = substrate conc
       xt(2) = x(2) + constants.dt*(-Fs/x(6)*x(2)+mygrowthrate); % C = cell conc
       xt(3) = x(3); % QO2 = OUR coefficient
       xt(4) = x(4) + constants.dt/constants.C_heat/x(6)*(constants.N_power*(w^3)+constants.Kq*x(3)*x(2)+(constants.Pp*Ip+(Ip^2)*constants.Rp)*constants.Np + constants.hA*(x(4)-x(5))); % Tc = culture temp
       xt(5) = x(5); % Tinf = environment temp
       xt(6) = x(6) + constants.dt*Fs;
       xt(7:8) = x(1:2);
       if constants.sample_interval > 1
           for j = 2:constants.sample_interval 
               xt(2*j+5:2*j+6) = x(2*j+3:2*j+4); % delayed states
           end
       end
    end

    function ypred = g(x)
        ypred = zeros(length(y),1);
        ypred(1) = constants.mf_in - x(3)*x(2)/Fg; % Measured mass fraction of O2 leaving system
        ypred(2) = 1 - 1/constants.mf_in*(1/Fg - 1/kLa/constants.pr)*x(3)*x(2); % Measured DO2
        ypred(3) = x(4); % Measured Tc
        ypred(4) = x(5); % measured Tinf
        ypred(5) = x(6);  % measured volume
        ypred(6:7) = x(end-1:end); % last two items in x are the most delayed
    end

    function mut = mu(S,C)
        mut = constants.mu_max*constants.Ki*S/(constants.Ki+S)/(constants.Ks+S)*C ;
    end
end

== matlab function Monod_delay_Controller/Bioreactor Dynamics/MATLAB Function1 ==
  data: x_in input; x_integrated input; xt output; constants parameter
function xt = delay_terms(x_in,x_integrated,constants)
       xt = zeros(size(x_in));
       xt(1:6) = x_integrated(1:6);
       if constants.sample_interval > 1
           for i = 2:constants.sample_interval 
               xt(2*i+5:2*i+6) = x_in(2*i+3:2*i+4); % delayed states
           end
       end
       xt(7:8) = x_in(1:2);
end
